simulink model "call_model"  (R2022a)
settings: Solver=ode113  StartTime=0.0  StopTime=1  RelTol=1e-5
values from neighbouring files (symbols this model uses):
  k = P_approx(1)    [firstlesson.m]
  Tm = P_approx(2)    [firstlesson.m]
  U = data(1,1)    [firstlesson.m]
settings Model: Creator=Xu  LastModifiedBy=Xu
settings SolverCC: ZeroCrossAlgorithm=Adaptive

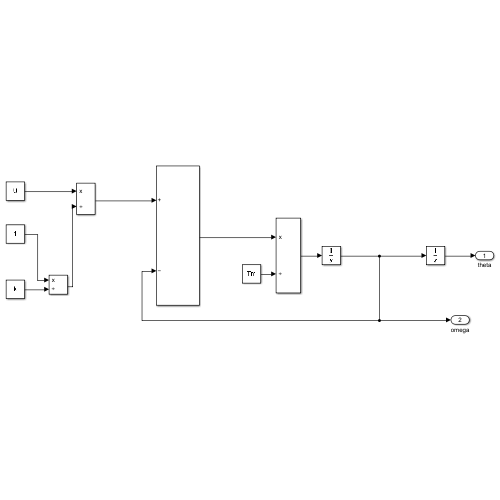
[thumbnail: Simulink's stored preview of the top-level diagram]
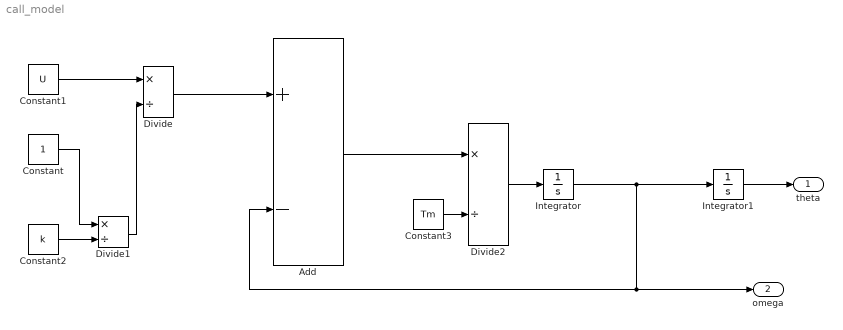
== system call_model ==
  Add : Sum  Inputs=+-
  Constant : Constant
  Constant1 : Constant  Value=U
  Constant2 : Constant  Value=k
  Constant3 : Constant  Value=Tm
  Divide : Product  Inputs=*/
  Divide1 : Product  Inputs=*/
  Divide2 : Product  Inputs=*/
  Integrator : Integrator
  Integrator1 : Integrator
  theta : Outport
  omega : Outport  Port=2
  wires:
  Divide1/1 -> Divide/2
  Constant1/1 -> Divide/1
  Constant2/1 -> Divide1/2
  Constant/1 -> Divide1/1
  Divide/1 -> Add/1
  Add/1 -> Divide2/1
  Constant3/1 -> Divide2/2
  Divide2/1 -> Integrator/1
  Integrator/1 -> omega/1, Add/2, Integrator1/1
  Integrator1/1 -> theta/1
